simulink model "trial"  (R2025b)
settings: Solver=VariableStepAuto  StartTime=0.0  StopTime=10.0  RelTol=1e-3
settings Model: Creator=l.sekules  LastModifiedBy=l.sekules

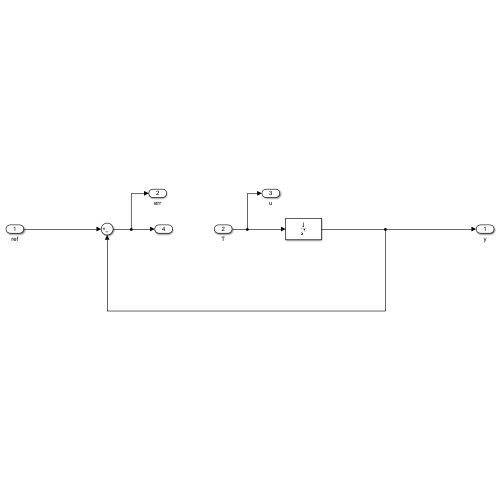
[thumbnail: Simulink's stored preview of the top-level diagram]
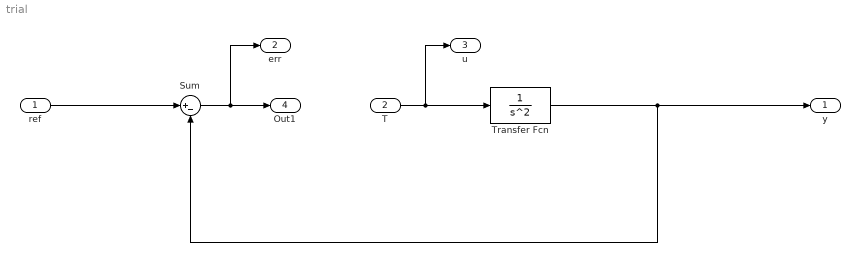
== system trial ==
  ref : Inport
  T : Inport  Port=2
  Sum : Sum  Inputs=|+-
  Transfer Fcn : TransferFcn  Denominator=[1 0 0]
  y : Outport
  err : Outport  Port=2
  u : Outport  Port=3
  Out1 : Outport  Port=4
  wires:
  ref/1 -> Sum/1
  Transfer Fcn/1 -> Sum/2, y/1
  Sum/1 -> Out1/1, err/1
  T/1 -> u/1, Transfer Fcn/1
